simulink model "sistem_2"  (R2026a)
settings: Solver=VariableStepAuto  StopTime=10
settings Model: Creator=ASUS  LastModifiedBy=ASUS

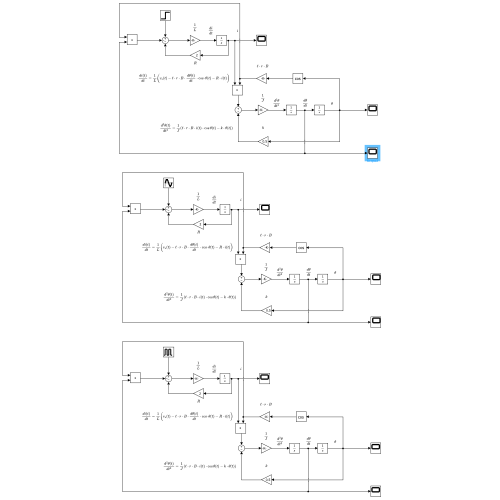
[thumbnail: Simulink's stored preview of the top-level diagram]
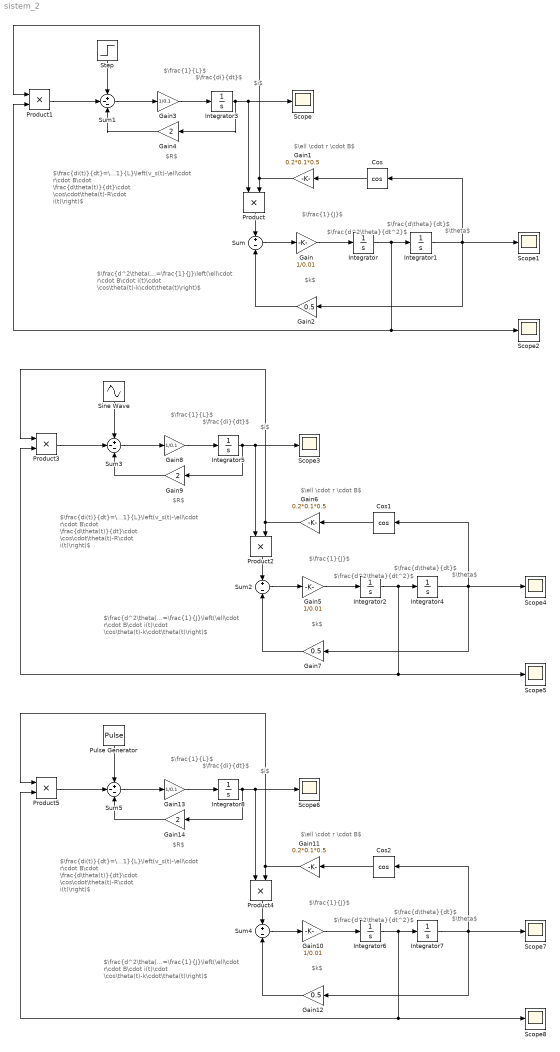
== system sistem_2 ==
  note: $\frac{di(t)}{dt}=\frac{1}{L}\left(v_s(t)-\ell\cdot r\cdot B\cdot \frac{d\theta(t)}{dt}\cdot \cos\cdot\theta(t)-R\cdot i(t)\right)$
  note: $\frac{1}{J}$
  note: $\ell \cdot r \cdot B$
  note: $\theta$
  note: $\frac{d\theta}{dt}$
  note: $\frac{d^2\theta}{dt^2}$
  note: $\frac{di}{dt}$
  note: $i$
  note: $k$
  note: $\frac{d^2\theta(t)}{dt^2}=\frac{1}{J}\left(\ell\cdot r\cdot B\cdot i(t)\cdot \cos\theta(t)-k\cdot\theta(t)\right)$
  note: $\frac{1}{L}$
  note: $R$
  note: $\frac{1}{J}$
  note: $\ell \cdot r \cdot B$
  note: $\theta$
  note: $\frac{di(t)}{dt}=\frac{1}{L}\left(v_s(t)-\ell\cdot r\cdot B\cdot \frac{d\theta(t)}{dt}\cdot \cos\cdot\theta(t)-R\cdot i(t)\right)$
  note: $\frac{d\theta}{dt}$
  note: $\frac{1}{L}$
  note: $\frac{d^2\theta(t)}{dt^2}=\frac{1}{J}\left(\ell\cdot r\cdot B\cdot i(t)\cdot \cos\theta(t)-k\cdot\theta(t)\right)$
  note: $k$
  note: $i$
  note: $\frac{d^2\theta}{dt^2}$
  note: $\frac{di}{dt}$
  note: $R$
  note: $\frac{1}{J}$
  note: $\ell \cdot r \cdot B$
  note: $\theta$
  note: $\frac{di(t)}{dt}=\frac{1}{L}\left(v_s(t)-\ell\cdot r\cdot B\cdot \frac{d\theta(t)}{dt}\cdot \cos\cdot\theta(t)-R\cdot i(t)\right)$
  note: $\frac{d\theta}{dt}$
  note: $\frac{1}{L}$
  note: $\frac{d^2\theta(t)}{dt^2}=\frac{1}{J}\left(\ell\cdot r\cdot B\cdot i(t)\cdot \cos\theta(t)-k\cdot\theta(t)\right)$
  note: $k$
  note: $i$
  note: $\frac{d^2\theta}{dt^2}$
  note: $\frac{di}{dt}$
  note: $R$
  Cos : Trigonometry  Operator=cos
  Cos1 : Trigonometry  Operator=cos
  Cos2 : Trigonometry  Operator=cos
  Gain : Gain  Gain=1/0.01
  Gain1 : Gain  Gain=0.2*0.1*0.5
  Gain10 : Gain  Gain=1/0.01
  Gain11 : Gain  Gain=0.2*0.1*0.5
  Gain12 : Gain  Gain=0.5
  Gain13 : Gain  Gain=1/0.1
  Gain14 : Gain  Gain=2
  Gain2 : Gain  Gain=0.5
  Gain3 : Gain  Gain=1/0.1
  Gain4 : Gain  Gain=2
  Gain5 : Gain  Gain=1/0.01
  Gain6 : Gain  Gain=0.2*0.1*0.5
  Gain7 : Gain  Gain=0.5
  Gain8 : Gain  Gain=1/0.1
  Gain9 : Gain  Gain=2
  Integrator{,2..3,5..6,8} (6 alike) : Integrator
  Integrator1 : Integrator  InitialCondition=0.1
  Integrator4 : Integrator  InitialCondition=0.1
  Integrator7 : Integrator  InitialCondition=0.1
  Product{,1..5} (6 alike) : Product
  Pulse Generator : DiscretePulseGenerator  PulseType=Time based  Amplitude=12  Period=10  PulseWidth=5
  Scope{,1..8} (9 alike) : Scope
      Scope settings: TimeSpan=10  ActiveDisplayYMinimum=-4.7854071925048407  ActiveDisplayYMaximum=11.605573498446679
      Scope1 settings: ActiveDisplayYMinimum=-0.14174569776201876  ActiveDisplayYMaximum=0.27648730309669484
      Scope2 settings: ActiveDisplayYMinimum=-1.0251214538677549  ActiveDisplayYMaximum=1.0253839305685459  DataLoggingVariableName=ScopeData2
      Scope3 settings: ActiveDisplayYMinimum=-1.5120071928423862  ActiveDisplayYMaximum=7.1804798255839657  DataLoggingVariableName=ScopeData3
      Scope4 settings: ActiveDisplayYMinimum=-0.28386436320709763  ActiveDisplayYMaximum=0.28539194377656024  DataLoggingVariableName=ScopeData4
      Scope5 settings: ActiveDisplayYMinimum=-1.0945599732566373  ActiveDisplayYMaximum=1.0874784940972904  DataLoggingVariableName=ScopeData5
      Scope6 settings: ActiveDisplayYMinimum=-1.5120071928423862  ActiveDisplayYMaximum=7.1804798255839657  DataLoggingVariableName=ScopeData6
      Scope7 settings: ActiveDisplayYMinimum=-0.14151990373054046  ActiveDisplayYMaximum=0.2745845605246936  DataLoggingVariableName=ScopeData7
      Scope8 settings: ActiveDisplayYMinimum=-1.0110640465386977  ActiveDisplayYMaximum=1.0120263226113118  DataLoggingVariableName=ScopeData8
  Sine Wave : Sin  Amplitude=12  SampleTime=0
  Step : Step  FinalValue=12  SampleTime=0
  Sum : Sum  Inputs=+-
  Sum1 : Sum  Inputs=+--
  Sum2 : Sum  Inputs=+-
  Sum3 : Sum  Inputs=+--
  Sum4 : Sum  Inputs=+-
  Sum5 : Sum  Inputs=+--
  wires:
  Integrator/1 -> Product1/2, Scope2/1, Integrator1/1
  Sum/1 -> Gain/1
  Gain/1 -> Integrator/1
  Integrator1/1 -> Gain2/1, Scope1/1, Cos/1
  Cos/1 -> Gain1/1
  Product/1 -> Sum/1
  Integrator3/1 -> Gain4/1, Scope/1, Product/1
  Gain1/1 -> Product1/1, Product/2
  Gain2/1 -> Sum/2
  Gain3/1 -> Integrator3/1
  Sum1/1 -> Gain3/1
  Step/1 -> Sum1/1
  Product1/1 -> Sum1/2
  Gain4/1 -> Sum1/3
  Gain5/1 -> Integrator2/1
  Integrator2/1 -> Product3/2, Scope5/1, Integrator4/1
  Sine Wave/1 -> Sum3/1
  Sum3/1 -> Gain8/1
  Integrator5/1 -> Gain9/1, Scope3/1, Product2/1
  Gain8/1 -> Integrator5/1
  Product2/1 -> Sum2/1
  Gain9/1 -> Sum3/3
  Gain7/1 -> Sum2/2
  Integrator4/1 -> Gain7/1, Scope4/1, Cos1/1
  Product3/1 -> Sum3/2
  Gain6/1 -> Product3/1, Product2/2
  Cos1/1 -> Gain6/1
  Sum2/1 -> Gain5/1
  Gain10/1 -> Integrator6/1
  Integrator6/1 -> Product5/2, Scope8/1, Integrator7/1
  Pulse Generator/1 -> Sum5/1
  Sum5/1 -> Gain13/1
  Integrator8/1 -> Gain14/1, Scope6/1, Product4/1
  Gain13/1 -> Integrator8/1
  Product4/1 -> Sum4/1
  Gain14/1 -> Sum5/3
  Gain12/1 -> Sum4/2
  Integrator7/1 -> Gain12/1, Scope7/1, Cos2/1
  Product5/1 -> Sum5/2
  Gain11/1 -> Product5/1, Product4/2
  Cos2/1 -> Gain11/1
  Sum4/1 -> Gain10/1
